simulink library "PoolIir"  (R2022b)
settings: Solver=VariableStepAuto  StartTime=0.0  StopTime=10.0  RelTol=1e-3
undefined symbols (not defined in the file or in its folder): Row
libraries: HandyTextFile x14, TuneVar x5, $bdroot x4, simulink x3, RTC x3, FeaturePath x2, TOP x2, AudioStats x1, CapturedConstLib x1
(part 2 of 2)

== matlab function PoolIir/PoolIirWithReset/PoolIirWithReset/SharcPlusAccelGxp/pooliir process ==
  data: x input; numStages input uint32; y output; coeffs input; codeWorkMemory data_store_memory
function y = pooliir_process(x, numStages, coeffs)
% Process function for Pooliir
%
% Parameters:
%   x:              input channels [frame size x number of inputs]
%   numStages:      coefficient sets [total filter lengths x 1]
%   coeffs:         array of filter lengths [number of filters x 1]
%
% Global parameters:
%   codeWorkMemory: working memory set up during roommode reset/init CRL
%                   function call [codeWorkMemorySize x 1]

% Extract configuration information from inputs
[frame_size, num_channels] = size(x);

% Initialize variables
global codeWorkMemory;

% Set correct data types
frame_size = uint32(frame_size);
num_channels = uint32(num_channels);

% Accelerator selection
if(coder.target('MATLAB') || coder.target('Sfun'))
    % Accelerator simulation
    y = pooliirAccel(x, frame_size, num_channels, numStages, coeffs);
else
    % Accelerator code generation
    y = iir_accelerator_process(x, codeWorkMemory);
end

end

function y = iir_accelerator_process(x, workMemory)
% If target == codegen, error out if no CRL found
coder.replace('-errorifnoreplacement');

[frameSize, numChannels]  = size(x);
y = zeros(frameSize, numChannels, 'single');
end

== matlab function PoolIir/PoolIirWithReset/PoolIirWithReset/SharcPlusAccelGxp/pooliir init ==
  data: x input; numStages input; coeffs input; codeWorkMemory data_store_memory; AccelDeviceId parameter
  events: trigger input FUNCTION_CALL_EVENT
function pooliir_init(x, numStages, coeffs, AccelDeviceId)
% Init function for Pooliir
%
% Parameters:
%   x:              input channels [frame size x number of inputs]
%   numStages:      coefficient sets [total filter lengths x 1]
%   coeffs:         array of filter lengths [number of filters x 1]
%
% Global parameters:
%   codeWorkMemory: working memory set up during roommode reset/init CRL
%                   function call [codeWorkMemorySize x 1]

%[Param:AccelDeviceId]

% Extract configuration information from inputs
[frame_size, num_channels] = size(x);

% Initialize variables
global codeWorkMemory;

% Get the work memory size
workMemorySize = numel(codeWorkMemory);

% Set correct data types
frame_size = uint32(frame_size);
num_channels = uint32(num_channels);
workMemorySize = uint32(workMemorySize);
AccelDeviceId = uint32(AccelDeviceId);
if(coder.target('MATLAB') || coder.target('Sfun'))
    return; % No init for simulation code
    
else
    % Call the Accel Init function
    y = pooliirAccelInit(x, frame_size, num_channels, numStages, coeffs, ...
        AccelDeviceId, codeWorkMemory, workMemorySize);

    % NOTE: The CRL mechanism requires an output for the function call,
    % and appears to be optimized out if that return value isn't used.
    % This is a dummy operation to make sure CRL ends up in generated code
    codeWorkMemory(1) = y;

end

end


function y = pooliirAccelInit(x, frame_size, num_channels, numStages, coeffs, ...
    accelDeviceId, workMemory, workMemorySize)
% If target == codegen, error out if no CRL found
coder.replace('-errorifnoreplacement');

% No init simulation code, but need to do something to ensure CRL does not
% get optimized out
y = workMemory(1) + 1;

end

== matlab function PoolIir/PoolIirWithReset/PoolIirWithReset/Generic/PoolIirProcess ==
  data: x input; numStages input uint32; y output single; coeffs input single; states data_store_memory
function y = pooliir_filter(x,numStages, coeffs)
%#codegen

% Extract configuration information from inputs
[frame_size, num_channels] = size(x);

% Initialize variables
global states;

% Typecast the variables
frame_size = uint32(frame_size);
num_channels = uint32(num_channels);

%Compute the filter coefficients
y = pooliir(x, frame_size, num_channels, numStages, coeffs, states);

end
